simulink model "Es2_sim"  (R2023b)
settings: Solver=VariableStepAuto  StartTime=0.0  StopTime=10.0  RelTol=1e-3
values from neighbouring files (symbols this model uses):
  x0 = [3;5]    [Es2.m]
settings Model: Creator=LENOVO  LastModifiedBy=LENOVO

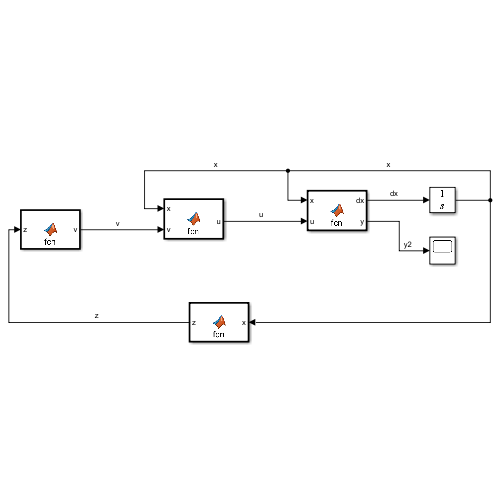
[thumbnail: Simulink's stored preview of the top-level diagram]
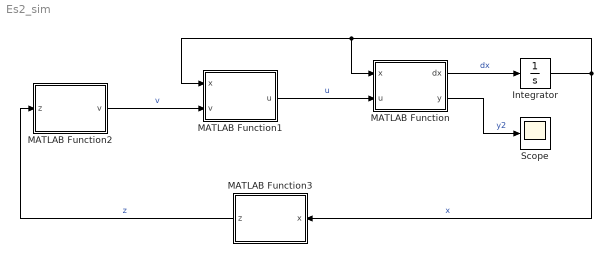
== system Es2_sim ==
  Integrator : Integrator  InitialCondition=x0
  MATLAB Function : MATLAB Function  TreatAsAtomicUnit=on
  MATLAB Function1 : MATLAB Function  TreatAsAtomicUnit=on
  MATLAB Function2 : MATLAB Function  TreatAsAtomicUnit=on
  MATLAB Function3 : MATLAB Function  TreatAsAtomicUnit=on
  Scope : Scope
  wires:
  MATLAB Function/1(dx) -> Integrator/1  "dx"
  Integrator/1 -> MATLAB Function3/1(x), MATLAB Function/1(x), MATLAB Function1/1(x)  "x"
  MATLAB Function1/1(u) -> MATLAB Function/2(u)  "u"
  MATLAB Function2/1(v) -> MATLAB Function1/2(v)  "v"
  MATLAB Function3/1(z) -> MATLAB Function2/1(z)  "z"
  MATLAB Function/2(y) -> Scope/1  "y2"

== matlab function Es2_sim/MATLAB Function ==
  data: x input; u input; dx output; y output
function [dx,y] = fcn(x,u)
X1=x(1);
X2=x(2);

dx = [X2*(3*X1^2 + 3*X1);X1 - 4*X2 + 3*u - X2*u];
y= 2*X1;

== matlab function Es2_sim/MATLAB Function2 ==
  data: z input; v output
function v = fcn(z)
Z1=z(1);
Z2=z(2);
k=[12.5;7.5];

v = -k(1)*Z1-k(2)*Z2;

== matlab function Es2_sim/MATLAB Function3 ==
  data: x input; z output
function z = fcn(x)
X1=x(1);
X2=x(2);
z = [2*X1 ; 2*X2*(3*X1 + 3*X1^2)];

== matlab function Es2_sim/MATLAB Function1 ==
  data: x input; u output; v input
function u = fcn(x,v)
X1=x(1);
X2=x(2);

u = ((6*X1 + 6*X1^2)*(X1 - 4*X2) - v + 2*X2^2*(6*X1 + 3)*(3*X1 + 3*X1^2))/((6*X1 + 6*X1^2)*(X2 - 3));
